simulink model "robot_floor"  (R2017b)
settings: Solver=ode15s  StartTime=0.0  StopTime=10.0  MaxStep=1e-2  RelTol=1e-4  AbsTol=1e-5
model workspace: external: MATLAB File D:\v6.1\Matlab\Robot\robot_DataFile.m (data not in the file)
undefined symbols (not defined in the file or in its folder): smiData, X, Y, Z
libraries: sm_lib x1864, nesl_utility x37, simulink x36, Contact_Forces_Lib x4
(part 37 of 37)

== matlab function robot_floor/Leg_model_left_1/leftFrontLegController/Subsystem/MATLAB Function1 ==
  data: kp input; kv input; x_desired input; dx_desired input; F input; T1 output; q1 input; q2 input; q3 input; x input; dx input; T2 output; T3 output
function [T1, T2, T3] = rightLegControl(kp, kv, x_desired, dx_desired, F, q1, q2, q3, x, dx)

g = [0     ;
     -9.8;
     0     ];

Mass_1 = [1.34705,  0,        0;
          0,        1.34705,  0;
          0,        0,        1.34705];

Iner_1 = [ 4228364.49e-09,     3044514.05e-09,    -301.13e-09;
           3044514.05e-09,    7122227.52e-09,     -208.78e-09;
           -301.13e-09,        -208.78e-09,       10540261.68e-09];

      
Mass_2 = [1.37462,  0,        0;
          0,        1.37462,  0;
          0,        0,        1.37462];

Iner_2 = [4320231.92e-09,     35.35e-09,           3693870.67e-09;
          35.35e-09,          13514184.12e-09,     -51.54e-09;
          3693870.67e-09,     -51.54e-09,          9829909.25e-09];

      
Mass_3 = [0.43648,  0,        0;
          0,        0.43648,  0;
          0,        0,        0.43648];
  
Iner_3 = [480014.29e-09,      -172.39e-09,        158.48e-09;
          -172.39e-09,        2763472.61e-09,     -3.33e-09;
          158.48e-09,         -3.33e-09,          2667913.18e-09];

      
Jv1 = [-0.05279*cos(q1)-0.12719*sin(q1),    0, 0;
       -0.05279*sin(q1)+0.12719*cos(q1),    0, 0;
       0,                                  0, 0];

Jw1 = [0, 0, 0;
       0, 0, 0;
       1, 0, 0];

   
Jv2 = [-0.14804*sin(q1)*cos(q2)-0.05166*cos(q1)-0.17*sin(q1),  -0.14804*cos(q1)*sin(q2),      0;
       0.14804*cos(q1)*cos(q2)-0.05166*sin(q1)+0.17*cos(q1),   -0.14804*sin(q1)*sin(q2),      0; 
       0,                                                      -0.14804*cos(q2),              0]; 
      
Jw2 = [0, -1, 0; 
       0,  0, 0; 
       1,  0, 0];
 
   
Jv3 = [-0.04483*sin(q1)*cos(q2-q3)-0.2*sin(q1)*cos(q2)-0.17*sin(q1),  -0.04483*cos(q1)*sin(q2-q3)-0.2*cos(q1)*sin(q2),  0.04483*cos(q1)*sin(q2-q3);
       0.04483*cos(q1)*cos(q2-q3)+0.2*cos(q1)*cos(q2)+0.17*cos(q1),   -0.04483*sin(q1)*sin(q2-q3)-0.2*sin(q1)*sin(q2),  0.04483*sin(q1)*sin(q2-q3);
       0,                                                             -0.04483*cos(q2-q3)-0.2*cos(q2),                  0.04483*cos(q2-q3)       ];
      
Jw3 = [0, -1, 1;
       0,  0, 0;
       1,  0, 0];

   
JvEE = [-0.245*sin(q1)*cos(q2-q3)-0.2*sin(q1)*cos(q2)-0.17*sin(q1),  -0.245*cos(q1)*sin(q2-q3)-0.2*cos(q1)*sin(q2),  0.245*cos(q1)*sin(q2-q3);
        0.245*cos(q1)*cos(q2-q3)+0.2*cos(q1)*cos(q2)+0.17*cos(q1),   -0.245*sin(q1)*sin(q2-q3)-0.2*sin(q1)*sin(q2),  0.245*sin(q1)*sin(q2-q3);
        0,                                                           -0.245*cos(q2-q3)-0.2*cos(q2),                  0.245*cos(q2-q3)       ];
   

Mass_q = Jv1'*Mass_1*Jv1 + Jw1'*Iner_1*Jw1 + Jv2'*Mass_2*Jv2 + Jw2'*Iner_2*Jw2 + Jv3'*Mass_3*Jv3 + Jw3'*Iner_3*Jw3;

Mass_x = JvEE'*pinv(JvEE*(inv(Mass_q))*JvEE');

Grav = Jv1'*Mass_1*g + Jv2'*Mass_2*g + Jv3'*Mass_3*g;

Force = JvEE'*F;

torque = Mass_x*((kp*(x_desired - x)) + (kv*(dx_desired - dx))) + Grav + Force;

T1 = torque(1);
T2 = torque(2);
T3 = torque(3);

== matlab function robot_floor/Leg_model_left_1/leftFrontLegController/Subsystem/MATLAB Function4 ==
  data: q1 input; x output; q2 input; q3 input
function x = Kinematics(q1, q2, q3)

leg = [0.245;
       0;
       0;
       1];
   
Trans0_3 = [cos(q1)*cos(q2-q3),    cos(q1)*sin(q2-q3),    sin(q1),       0.2*cos(q1)*cos(q2)+0.17*cos(q1);
            sin(q1)*cos(q2-q3),    sin(q1)*sin(q2-q3),    -cos(q1),      0.2*sin(q1)*cos(q2)+0.17*sin(q1);
            -sin(q2-q3),           cos(q2-q3),            0,             -0.2*sin(q2);
            0,                      0,                    0,              1];
        
x_temp = Trans0_3*leg;

x = x_temp(1:3);

== matlab function robot_floor/Leg_model_left_1/leftFrontLegController/Subsystem/MATLAB Function5 ==
  data: q1 input; dx output; q2 input; q3 input; dq1 input; dq2 input; dq3 input
function dx = Jacobian(q1, q2, q3, dq1, dq2, dq3)

dq = [ dq1;
       dq2;
       dq3];

JvEE = [-0.245*sin(q1)*cos(q2-q3)-0.2*sin(q1)*cos(q2)-0.17*sin(q1),  -0.245*cos(q1)*sin(q2-q3)-0.2*cos(q1)*sin(q2),  0.245*cos(q1)*sin(q2-q3);
        0.245*cos(q1)*cos(q2-q3)+0.2*cos(q1)*cos(q2)+0.17*cos(q1),   -0.245*sin(q1)*sin(q2-q3)-0.2*sin(q1)*sin(q2),  0.245*sin(q1)*sin(q2-q3);
        0,                                                           -0.245*cos(q2-q3)-0.2*cos(q2),                  0.245*cos(q2-q3)       ];
   
dx = JvEE*dq;

== matlab function robot_floor/Leg_model_right_2/leftRearLegController /MATLAB Function ==
  data: in1 input; out output; in2 input; in3 input
function out = matrix(in1, in2, in3)
out = [in1; in2; in3];

== matlab function robot_floor/Leg_model_right_2/leftRearLegController /MATLAB Function1 ==
  data: in1 input; out output; in2 input; in3 input
function out = matrix(in1, in2, in3)
out = [in1; in2; in3];

== matlab function robot_floor/Leg_model_right_2/leftRearLegController /MATLAB Function2 ==
  data: in1 input; out output; in2 input; in3 input
function out = matrix(in1, in2, in3)
out = [in1; in2; in3];

== matlab function robot_floor/Leg_model_right_2/leftRearLegController /Subsystem/MATLAB Function1 ==
  data: kp input; kv input; x_desired input; dx_desired input; F input; T1 output; q1 input; q2 input; q3 input; x input; dx input; T2 output; T3 output
function [T1, T2, T3] = rightLegControl(kp, kv, x_desired, dx_desired, F, q1, q2, q3, x, dx)

g = [0     ;
     -9.8;
     0     ];

Mass_1 = [1.34705,  0,        0;
          0,        1.34705,  0;
          0,        0,        1.34705];

Iner_1 = [ 4228364.49e-09,      -3044514.05e-09,     212.52e-09;
           -3044408.99e-09,     7121809.49e-09,     -363.95e-09;
           212.52e-09,          -363.95e-09,         10539827.01e-09];

      
Mass_2 = [1.37462,  0,        0;
          0,        1.37462,  0;
          0,        0,        1.37462];

Iner_2 = [4320221.32e-09,      -231.05e-09,        -3693903.88e-09;
          -231.05e-09,         13514346.24e-09,     8.54e-09;
          -3693903.88e-09,     8.54e-09,            9830060.78e-09];

      
Mass_3 = [0.43648,  0,        0;
          0,        0.43648,  0;
          0,        0,        0.43648];
  
Iner_3 = [480002.60e-09,      -172.39e-09,        158.48e-09;
          -172.39e-09,        2763460.92e-09,     -3.33e-09;
          158.48e-09,         -3.33e-09,          2667913.18e-09];

      
Jv1 = [0.05279*cos(q1)-0.12719*sin(q1),    0, 0;
       0.05279*sin(q1)+0.12719*cos(q1),    0, 0;
       0,                                  0, 0];

Jw1 = [0, 0, 0;
       0, 0, 0;
       1, 0, 0];

   
Jv2 = [-0.14804*sin(q1)*cos(q2)+0.05166*cos(q1)-0.17*sin(q1),  -0.14804*cos(q1)*sin(q2),      0;
       0.14804*cos(q1)*cos(q2)+0.05166*sin(q1)+0.17*cos(q1),   -0.14804*sin(q1)*sin(q2),      0; 
       0,                                                      -0.14804*cos(q2),              0]; 
      
Jw2 = [0, -1, 0; 
       0,  0, 0; 
       1,  0, 0];
 
   
Jv3 = [-0.04483*sin(q1)*cos(q2-q3)-0.2*sin(q1)*cos(q2)-0.17*sin(q1),  -0.04483*cos(q1)*sin(q2-q3)-0.2*cos(q1)*sin(q2),  0.04483*cos(q1)*sin(q2-q3);
       0.04483*cos(q1)*cos(q2-q3)+0.2*cos(q1)*cos(q2)+0.17*cos(q1),   -0.04483*sin(q1)*sin(q2-q3)-0.2*sin(q1)*sin(q2),  0.04483*sin(q1)*sin(q2-q3);
       0,                                                             -0.04483*cos(q2-q3)-0.2*cos(q2),                  0.04483*cos(q2-q3)       ];
      
Jw3 = [0, -1, 1;
       0,  0, 0;
       1,  0, 0];

   
JvEE = [-0.245*sin(q1)*cos(q2-q3)-0.2*sin(q1)*cos(q2)-0.17*sin(q1),  -0.245*cos(q1)*sin(q2-q3)-0.2*cos(q1)*sin(q2),  0.245*cos(q1)*sin(q2-q3);
        0.245*cos(q1)*cos(q2-q3)+0.2*cos(q1)*cos(q2)+0.17*cos(q1),   -0.245*sin(q1)*sin(q2-q3)-0.2*sin(q1)*sin(q2),  0.245*sin(q1)*sin(q2-q3);
        0,                                                           -0.245*cos(q2-q3)-0.2*cos(q2),                  0.245*cos(q2-q3)       ];
   

Mass_q = Jv1'*Mass_1*Jv1 + Jw1'*Iner_1*Jw1 + Jv2'*Mass_2*Jv2 + Jw2'*Iner_2*Jw2 + Jv3'*Mass_3*Jv3 + Jw3'*Iner_3*Jw3;

Mass_x = JvEE'*pinv(JvEE*(inv(Mass_q))*JvEE');

Grav = Jv1'*Mass_1*g + Jv2'*Mass_2*g + Jv3'*Mass_3*g;

Force = JvEE'*F;

torque = Mass_x*((kp*(x_desired - x)) + (kv*(dx_desired - dx))) + Grav + Force;

T1 = torque(1);
T2 = torque(2);
T3 = torque(3);

== matlab function robot_floor/Leg_model_right_2/leftRearLegController /Subsystem/MATLAB Function4 ==
  data: q1 input; x output; q2 input; q3 input
function x = Kinematics(q1, q2, q3)

leg = [0.245;
       0;
       0;
       1];
   
Trans0_3 = [cos(q1)*cos(q2-q3),    cos(q1)*sin(q2-q3),    sin(q1),       0.2*cos(q1)*cos(q2)+0.17*cos(q1);
            sin(q1)*cos(q2-q3),    sin(q1)*sin(q2-q3),    -cos(q1),      0.2*sin(q1)*cos(q2)+0.17*sin(q1);
            -sin(q2-q3),           cos(q2-q3),            0,             -0.2*sin(q2);
            0,                      0,                    0,              1];
        
x_temp = Trans0_3*leg;

x = x_temp(1:3);

== matlab function robot_floor/Leg_model_right_2/leftRearLegController /Subsystem/MATLAB Function5 ==
  data: q1 input; dx output; q2 input; q3 input; dq1 input; dq2 input; dq3 input
function dx = Jacobian(q1, q2, q3, dq1, dq2, dq3)

dq = [ dq1;
       dq2;
       dq3];

JvEE = [-0.245*sin(q1)*cos(q2-q3)-0.2*sin(q1)*cos(q2)-0.17*sin(q1),  -0.245*cos(q1)*sin(q2-q3)-0.2*cos(q1)*sin(q2),  0.245*cos(q1)*sin(q2-q3);
        0.245*cos(q1)*cos(q2-q3)+0.2*cos(q1)*cos(q2)+0.17*cos(q1),   -0.245*sin(q1)*sin(q2-q3)-0.2*sin(q1)*sin(q2),  0.245*sin(q1)*sin(q2-q3);
        0,                                                           -0.245*cos(q2-q3)-0.2*cos(q2),                  0.245*cos(q2-q3)       ];
   
dx = JvEE*dq;

== matlab function robot_floor/Leg_model_left_2/rightRearLegController /MATLAB Function ==
  data: in1 input; out output; in2 input; in3 input
function out = matrix(in1, in2, in3)
out = [in1; in2; in3];

== matlab function robot_floor/Leg_model_left_2/rightRearLegController /MATLAB Function1 ==
  data: in1 input; out output; in2 input; in3 input
function out = matrix(in1, in2, in3)
out = [in1; in2; in3];

== matlab function robot_floor/Leg_model_left_2/rightRearLegController /MATLAB Function2 ==
  data: in1 input; out output; in2 input; in3 input
function out = matrix(in1, in2, in3)
out = [in1; in2; in3];

== matlab function robot_floor/Leg_model_left_2/rightRearLegController /Subsystem/MATLAB Function1 ==
  data: kp input; kv input; x_desired input; dx_desired input; F input; T1 output; q1 input; q2 input; q3 input; x input; dx input; T2 output; T3 output
function [T1, T2, T3] = rightLegControl(kp, kv, x_desired, dx_desired, F, q1, q2, q3, x, dx)

g = [0     ;
     -9.8;
     0     ];

Mass_1 = [1.34705,  0,        0;
          0,        1.34705,  0;
          0,        0,        1.34705];

Iner_1 = [ 4228364.49e-09,      3044514.05e-09,     -285.87e-09;
           3044514.05e-09,      7122227.52e-09,     -208.78e-09;
           -285.87e-09,         -208.78e-09,        10540261.68e-09];

      
Mass_2 = [1.37462,  0,        0;
          0,        1.37462,  0;
          0,        0,        1.37462];

Iner_2 = [4320231.92e-09,     -130.56e-09,          3693870.67e-09;
          -130.56e-09,        13514184.12e-09,     -51.54e-09;
          3693870.67e-09,     -51.54e-09,           9829909.25e-09];

      
Mass_3 = [0.43648 ,  0,        0;
          0,        0.43648,  0;
          0,        0,        0.43648];
  
Iner_3 = [480014.29e-09,     -76.38e-09,       -3666.08e-09;
          -76.38e-09,        2763472.61e-09,   -3.33e-09;
          -3666.08e-09,      -3.33e-09,        2667913.18e-09];

      
Jv1 = [-0.05279*cos(q1)-0.12719*sin(q1),    0, 0;
       -0.05279*sin(q1)+0.12719*cos(q1),    0, 0;
       0,                                  0, 0];

Jw1 = [0, 0, 0;
       0, 0, 0;
       1, 0, 0];

   
Jv2 = [-0.14804*sin(q1)*cos(q2)-0.05166*cos(q1)-0.17*sin(q1),  -0.14804*cos(q1)*sin(q2),      0;
        0.14804*cos(q1)*cos(q2)-0.05166*sin(q1)+0.17*cos(q1),  -0.14804*sin(q1)*sin(q2),      0; 
        0,                                                     -0.09947*cos(q2),              0]; 
      
Jw2 = [0, -1, 0; 
       0,  0, 0; 
       1,  0, 0];
 
   
Jv3 = [-0.04483*sin(q1)*cos(q2-q3)-0.2*sin(q1)*cos(q2)-0.17*sin(q1),  -0.04483*cos(q1)*sin(q2-q3)-0.2*cos(q1)*sin(q2),  0.03084*cos(q1)*sin(q2-q3);
       0.04483*cos(q1)*cos(q2-q3)+0.2*cos(q1)*cos(q2)+0.17*cos(q1),   -0.04483*sin(q1)*sin(q2-q3)-0.2*sin(q1)*sin(q2),  0.03084*sin(q1)*sin(q2-q3);
       0,                                                             -0.04483*cos(q2-q3)-0.2*cos(q2),                  0.03084*cos(q2-q3)];
      
Jw3 = [0, -1, 1;
       0,  0, 0;
       1,  0, 0];

   
JvEE = [-0.245*sin(q1)*cos(q2-q3)-0.2*sin(q1)*cos(q2)-0.17*sin(q1),  -0.245*cos(q1)*sin(q2-q3)-0.2*cos(q1)*sin(q2),  0.245*cos(q1)*sin(q2-q3);
        0.245*cos(q1)*cos(q2-q3)+0.2*cos(q1)*cos(q2)+0.17*cos(q1),   -0.245*sin(q1)*sin(q2-q3)-0.2*sin(q1)*sin(q2),  0.245*sin(q1)*sin(q2-q3);
        0,                                                           -0.245*cos(q2-q3)-0.2*cos(q2),                  0.245*cos(q2-q3)       ];
   

Mass_q = Jv1'*Mass_1*Jv1 + Jw1'*Iner_1*Jw1 + Jv2'*Mass_2*Jv2 + Jw2'*Iner_2*Jw2 + Jv3'*Mass_3*Jv3 + Jw3'*Iner_3*Jw3;

Mass_x = JvEE'*pinv(JvEE*(inv(Mass_q))*JvEE');

Grav = Jv1'*Mass_1*g + Jv2'*Mass_2*g + Jv3'*Mass_3*g;

Force = JvEE'*F;

torque = Mass_x*((kp*(x_desired - x)) + (kv*(dx_desired - dx))) + Grav + Force;

T1 = torque(1);
T2 = torque(2);
T3 = torque(3);

== matlab function robot_floor/Leg_model_left_2/rightRearLegController /Subsystem/MATLAB Function4 ==
  data: q1 input; x output; q2 input; q3 input
function x = Kinematics(q1, q2, q3)

leg = [0.245;
       0;
       0;
       1];
   
Trans0_3 = [cos(q1)*cos(q2-q3),    cos(q1)*sin(q2-q3),    sin(q1),       0.2*cos(q1)*cos(q2)+0.17*cos(q1);
            sin(q1)*cos(q2-q3),    sin(q1)*sin(q2-q3),    -cos(q1),      0.2*sin(q1)*cos(q2)+0.17*sin(q1);
            -sin(q2-q3),           cos(q2-q3),            0,             -0.2*sin(q2);
            0,                      0,                    0,              1];
        
x_temp = Trans0_3*leg;

x = x_temp(1:3);

== matlab function robot_floor/Leg_model_left_2/rightRearLegController /Subsystem/MATLAB Function5 ==
  data: q1 input; dx output; q2 input; q3 input; dq1 input; dq2 input; dq3 input
function dx = Jacobian(q1, q2, q3, dq1, dq2, dq3)

dq = [ dq1;
       dq2;
       dq3];

JvEE = [-0.245*sin(q1)*cos(q2-q3)-0.2*sin(q1)*cos(q2)-0.17*sin(q1),  -0.245*cos(q1)*sin(q2-q3)-0.2*cos(q1)*sin(q2),  0.245*cos(q1)*sin(q2-q3);
        0.245*cos(q1)*cos(q2-q3)+0.2*cos(q1)*cos(q2)+0.17*cos(q1),   -0.245*sin(q1)*sin(q2-q3)-0.2*sin(q1)*sin(q2),  0.245*sin(q1)*sin(q2-q3);
        0,                                                           -0.245*cos(q2-q3)-0.2*cos(q2),                  0.245*cos(q2-q3)       ];
   
dx = JvEE*dq;
